simulink library "lib_transmission2"  (Simulink 4.1.1)
values from neighbouring files (symbols this model uses):
  logFlag = 1    [advSACompMaskInit.m]    (also in advSACompMaskInitR13.m)
undefined symbols (not defined in the file or in its folder): cyc_mph, fc_map_spd, fc_max_trq, fc_spd_scale, fc_trq_scale, fd_inertia, fd_loss, fd_ratio, gb_dnshift_load, gb_dnshift_spd, gb_gear_number_lookup, gb_gears_num, gb_inertia, gb_loss_const, gb_loss_input_spd_coeff, gb_loss_input_trq_coeff, gb_loss_output_spd_coeff, gb_loss_output_trq_coeff, gb_map_spd_out, gb_map_trq_in, gb_map_trq_out, gb_num_init, gb_ratio, gb_shift_delay, gb_spd_scale, gb_trq_scale, gb_upshift_load, gb_upshift_spd, htc_inertia, htc_k_adv, htc_k_adv_coast, htc_lockup, htc_lockup_load, htc_lockup_spd, htc_lu_gear_range, htc_max_coast_tr, htc_min_coast_tr, htc_pump_loss_spd, htc_pump_loss_trq_lockup, htc_pump_loss_trq_unlock, htc_sr, htc_sr_coast, htc_tr, htc_tr_coast, htc_unlock_spd, mc_map_spd, mc_max_trq, mc_overtrq_factor, mc_spd_scale, mc_trq_scale, tc_loss, tc_mc_to_fc_ratio, tx_eff_map, tx_map_spd, tx_map_trq, tx_pg_r, tx_pg_s, tx_speed_dep, vc_clutch_bool, vc_idle_spd ... (+2)
libraries: lib_controls x1, lib_etc x1, lib_controls2 x1, lib_transmission x1
(part 16 of 17)

== system lib_transmission2/Gearbox Control/automatic transmission gearbox and htc standard lockup logic for htc shift logic for gearbox/gearbox control for use w/ AT/shifting1/time since last shift ==
  in_1 : Inport  Port=1  LatchInput=off
  just shifted : Subsystem
      settings: RTWFcnNameOpts=Auto  RTWFileNameOpts=Auto
      mask Display: disp('just\nshifted')
  timer : Subsystem
      settings: RTWFcnNameOpts=Auto  RTWFileNameOpts=Auto
      mask Display: disp('timer')
  out_1 : Outport  Port=1  InitialOutput=0
  wires:
  timer/1(time) -> out_1/1
  just shifted/1(out_1) -> timer/1(trigger)
  in_1/1 -> just shifted/1(in_1)

== system lib_transmission2/Gearbox Control/automatic transmission gearbox and htc standard lockup logic for htc shift logic for gearbox/gearbox control for use w/ AT/upshift  command/load fraction ==
  In1 : Inport  Port=1  LatchInput=off
  S-Function : S-Function  FunctionName=sfun_gearbox  Parameters=load, spd  PortCounts=[]  SFunctionModules=''
  Out1 : Outport  Port=1  InitialOutput=0
  wires:
  In1/1 -> S-Function/1
  S-Function/1 -> Out1/1

== system lib_transmission2/Gearbox Control/time lookup shift logic for gearbox/lookup/shifting determination/time since last shift ==
  in_1 : Inport  Port=1  LatchInput=off
  just shifted : Subsystem
      settings: RTWFcnNameOpts=Auto  RTWFileNameOpts=Auto
      mask Display: disp('just\nshifted')
  timer : Subsystem
      settings: RTWFcnNameOpts=Auto  RTWFileNameOpts=Auto
      mask Display: disp('timer')
  out_1 : Outport  Port=1  InitialOutput=0
  wires:
  timer/1(time) -> out_1/1
  just shifted/1(out_1) -> timer/1(trigger)
  in_1/1 -> just shifted/1(in_1)

== system lib_transmission2/Gearbox Control/vehicle speed dependent shift logic for gearbox/speed dependent/Speed Dependent Shifting/shifting ==
  gear number : Inport  Port=1  LatchInput=off
  Constant : Constant  Value=gb_shift_delay-1e-6
  Relational Operator : RelationalOperator  Operator=<
  time since last shift : Subsystem
      settings: RTWFcnNameOpts=Auto  RTWFileNameOpts=Auto
      mask Display: disp('time since\nlast shift')
  out_1 : Outport  Port=1  InitialOutput=0
  wires:
  time since last shift/1(out_1) -> Relational Operator/1
  Constant/1 -> Relational Operator/2
  gear number/1 -> time since last shift/1(in_1)
  Relational Operator/1 -> out_1/1

== system lib_transmission2/Gearbox Control/vehicle speed dependent shift logic for gearbox/speed dependent/Speed Dependent Shifting/shifting1 ==
  gear number : Inport  Port=1  LatchInput=off
  Constant : Constant  Value=gb_shift_delay-1e-6
  Relational Operator : RelationalOperator  Operator=<
  time since last shift : Subsystem
      settings: RTWFcnNameOpts=Auto  RTWFileNameOpts=Auto
      mask Display: disp('time since\nlast shift')
  out_1 : Outport  Port=1  InitialOutput=0
  wires:
  time since last shift/1(out_1) -> Relational Operator/1
  Constant/1 -> Relational Operator/2
  gear number/1 -> time since last shift/1(in_1)
  Relational Operator/1 -> out_1/1

== system lib_transmission2/gearbox <gb>/gearbox model & interface/gearbox model/Pout/Pin neglecting inertia/Pout/Pin (neglecting inertia) ==
  in_1 : Inport  Port=1  LatchInput=off
  in_2 : Inport  Port=2  LatchInput=off
  Fcn : Fcn  Expr=1/u
  Product : Product  Inputs=2  Multiplication=Element-wise(.*)  SaturateOnIntegerOverflow=on
  out_1 : Outport  Port=1  InitialOutput=0
  wires:
  in_2/1 -> Fcn/1
  Product/1 -> out_1/1
  Fcn/1 -> Product/2
  in_1/1 -> Product/1

== system lib_transmission2/gearbox <gb>/gearbox model & interface/gearbox model/Pout/Pin neglecting inertia/make division bombproof ==
  note: only add eps if Tin-Tinertia is == 0 (this avoids problems when Tin-Tineratia == -eps
      | which happens from time to time
  Tin-Tinertia : Inport  Port=1  LatchInput=off
  Block NOTES : Subsystem
      settings: RTWFcnNameOpts=Auto  RTWFileNameOpts=Auto
      mask Display: disp('Block\nNOTES')
  Constant : Constant  Orientation=up  Value=eps
  Constant1 : Constant  Orientation=up  Value=0
  Product : Product  Inputs=2  Multiplication=Element-wise(.*)  SaturateOnIntegerOverflow=on
  Relational Operator1 : RelationalOperator  Operator===
  make division bombproof : Sum  Inputs=++  SaturateOnIntegerOverflow=on
  Out1 : Outport  Port=1
  wires:
  make division bombproof/1 -> Out1/1
  Constant/1 -> Product/2
  Relational Operator1/1 -> Product/1
  Product/1 -> make division bombproof/2
  Constant1/1 -> Relational Operator1/2
  Tin-Tinertia/1 -> Relational Operator1/1, make division bombproof/1

== system lib_transmission2/gearbox <gb>/gearbox model & interface/gearbox model/gearbox controller interface/enhancedToWorkspace1 ==
  In1 : Inport  Port=1  LatchInput=off
  To Workspace : ToWorkspace  VariableName=gb_gear_ratio  SampleTime=-1  SaveFormat=Array
  wires:
  In1/1 -> To Workspace/1

== system lib_transmission2/gearbox <gb>/gearbox model & interface/gearbox model/gearbox controller interface/enhancedToWorkspace8 ==
  In1 : Inport  Port=1  LatchInput=off
  To Workspace : ToWorkspace  VariableName=gb_shifting  SampleTime=-1  SaveFormat=Array
  wires:
  In1/1 -> To Workspace/1

== system lib_transmission2/gearbox <gb>/gearbox model & interface/gearbox model/loss (Nm)/3D discrete lookup table (sfun) ==
  lookup speed (rad/s) : Inport  Port=1  LatchInput=off
  lookup trq (Nm) : Inport  Port=2  LatchInput=off
  "gear_number  (e.g., 1, 2, 3)" : Inport  Port=3  LatchInput=off
  Mux : Mux  Inputs=3
  Saturation : Saturate  UpperLimit=max(tx_map_spd)  LowerLimit=min(tx_map_spd)  LinearizeAsGain=on
  Saturation1 : Saturate  UpperLimit=max(tx_map_trq)  LowerLimit=min(tx_map_trq)  LinearizeAsGain=on
  Saturation2 : Saturate  UpperLimit=size(tx_eff_map,3)  LowerLimit=1  LinearizeAsGain=on
  discrete interp2d : S-Function  FunctionName=sfun_discreteLookup3d  Parameters=tx_map_trq, tx_map_spd, tx_eff_map  PortCounts=[]  SFunctionModules=''
  tx_eff : Outport  Port=1
  wires:
  discrete interp2d/1 -> tx_eff/1
  Mux/1 -> discrete interp2d/1
  lookup speed (rad/s)/1 -> Saturation/1
  Saturation/1 -> Mux/1
  lookup trq (Nm)/1 -> Saturation1/1
  Saturation1/1 -> Mux/2
  "gear_number  (e.g., 1, 2, 3)"/1 -> Saturation2/1
  Saturation2/1 -> Mux/3

== system lib_transmission2/gearbox <gb>/gearbox model & interface/gearbox model/loss (Nm)/Block NOTES ==
  note: 5 July 2001:mpo changing loss block to a lookup table methodology
      | 12/20/00:tm revised loss saturation block. lower limit changed
      | from 1 to 0 and upper limit changed from 100 to inf to prevent over or under penalties
  note: Revision Notes:

== system lib_transmission2/gearbox <gb>/gearbox model & interface/gearbox model/loss (Nm)/enhancedToWorkspace ==
  In1 : Inport  Port=1  LatchInput=off
  To Workspace : ToWorkspace  VariableName=gb_current_gear_ratio  SampleTime=-1  SaveFormat=Array
  wires:
  In1/1 -> To Workspace/1

== system lib_transmission2/gearbox <gb>/gearbox model & interface/gearbox model/loss (Nm)/enhancedToWorkspace1 ==
  In1 : Inport  Port=1  LatchInput=off
  To Workspace : ToWorkspace  VariableName=gb_spin_loss_trq  SampleTime=-1  SaveFormat=Array
  wires:
  In1/1 -> To Workspace/1

== system lib_transmission2/gearbox <gb> CVT/CVT model & interface/CVT gearbox  <gb>/gearbox  efficiency/enhancedToWorkspace ==
  In1 : Inport  Port=1  LatchInput=off
  Terminator : Terminator
  wires:
  In1/1 -> Terminator/1

== system lib_transmission2/gearbox <gb> CVT/CVT model & interface/CVT gearbox  <gb>/loss (Nm)/Input Torque: 3-D interpolation ==
  output torque (N*m) : Inport  Port=1  LatchInput=off
  output speed (rad/s) : Inport  Port=2  LatchInput=off
  pulley ratio : Inport  Port=3  LatchInput=off
  Constant3 : Constant  Value=eps
  Constant4 : Constant  Value=0
  Demux2 : Demux  Outputs=2  BusSelectionMode=off
  Look-Up Table1 : Lookup  InputValues=[1:max(size(gb_ratio))]  OutputValues=gb_ratio
  Look-Up Table2 : Lookup  InputValues=[1:max(size(gb_ratio))]  OutputValues=gb_ratio
  Mux1 : Mux  Inputs=4
      settings: DisplayOption=none
  Mux2 : Mux  Inputs=3
      settings: DisplayOption=none
  Mux3 : Mux  Inputs=2
      settings: DisplayOption=none
  Mux4 : Mux  Inputs=2
      settings: DisplayOption=none
  Mux7 : Mux  Inputs=4
      settings: DisplayOption=none
  Product1 : Product  Inputs=3  Multiplication=Element-wise(.*)  SaturateOnIntegerOverflow=on
  Product2 : Product  Inputs=*//  Multiplication=Element-wise(.*)  SaturateOnIntegerOverflow=on
  Sum2 : Sum  Inputs=2  SaturateOnIntegerOverflow=on
  Switch1 : Switch  Threshold=eps
  indices of nearest pulley ratios for which there exist maps : Subsystem
      settings: RTWFcnNameOpts=Auto  RTWFileNameOpts=Auto
  linear eqn for power : Fcn  Expr=u[5]*(u[6]-u[3])+u[1]
  slope for linear interp. : Fcn  Expr=(u[1]-u[2])/(u[3]-u[4]+eps)
  trq in  look-up : Subsystem  mask{P1=gb_map_spd_out*gb_spd_scale, P2=gb_map_trq_in*gb_trq_scale, P3=gb_map_trq_out*gb_trq_scale, P4=gb_ratio}
      mask prompts: P1 "Vector of output speeds"; P2 "Vector of input torques"; P3 "Table of output torques"; P4 "Vector of gear ratios"
      settings: RTWFcnNameOpts=Auto  RTWFileNameOpts=Auto
  input torque (Nm) : Outport  Port=1  InitialOutput=0
  wires:
  pulley ratio/1 -> indices of nearest pulley ratios for which there exist maps/1(in_1), Mux2/3, Product2/3
  indices of nearest pulley ratios for which there exist maps/1(index of upper bounding map) -> Look-Up Table1/1, Mux7/3
  indices of nearest pulley ratios for which there exist maps/2(index of lower bounding map) -> Look-Up Table2/1, Mux7/4
  Mux7/1 -> trq in  look-up/1(In1)
  slope for linear interp./1 -> Mux2/2
  Mux2/1 -> linear eqn for power/1
  Mux1/1 -> Mux2/1, slope for linear interp./1
  Demux2/2 -> Mux1/2
  output torque (N*m)/1 -> Mux7/1
  Demux2/1 -> Mux1/1
  Look-Up Table1/1 -> Mux1/3, Mux3/1
  Look-Up Table2/1 -> Mux1/4, Mux3/2
  output speed (rad/s)/1 -> Mux7/2, Mux4/1, Mux4/2, Sum2/1, Switch1/2
  trq in  look-up/1(Out1) -> Product1/2
  Mux4/1 -> Product1/1
  Mux3/1 -> Product1/3
  Product1/1 -> Demux2/1
  linear eqn for power/1 -> Product2/1
  Sum2/1 -> Product2/2
  Product2/1 -> Switch1/1
  Switch1/1 -> input torque (Nm)/1
  Constant4/1 -> Switch1/3
  Constant3/1 -> Sum2/2

== system lib_transmission2/gearbox <gb> old/gearbox model & interface/gearbox model/Pout/Pin neglecting inertia/Pout/Pin (neglecting inertia) ==
  in_1 : Inport  Port=1  LatchInput=off
  in_2 : Inport  Port=2  LatchInput=off
  Fcn : Fcn  Expr=1/u
  Product : Product  Inputs=2  Multiplication=Element-wise(.*)  SaturateOnIntegerOverflow=on
  out_1 : Outport  Port=1  InitialOutput=0
  wires:
  in_2/1 -> Fcn/1
  Product/1 -> out_1/1
  Fcn/1 -> Product/2
  in_1/1 -> Product/1

== system lib_transmission2/gearbox <gb> old/gearbox model & interface/gearbox model/Pout/Pin neglecting inertia/make division bombproof ==
  note: only add eps if Tin-Tinertia is == 0 (this avoids problems when Tin-Tineratia == -eps
      | which happens from time to time
  Tin-Tinertia : Inport  Port=1  LatchInput=off
  Block NOTES : Subsystem
      settings: RTWFcnNameOpts=Auto  RTWFileNameOpts=Auto
      mask Display: disp('Block\nNOTES')
  Constant : Constant  Orientation=up  Value=eps
  Constant1 : Constant  Orientation=up  Value=0
  Product : Product  Inputs=2  Multiplication=Element-wise(.*)  SaturateOnIntegerOverflow=on
  Relational Operator1 : RelationalOperator  Operator===
  make division bombproof : Sum  Inputs=++  SaturateOnIntegerOverflow=on
  Out1 : Outport  Port=1
  wires:
  make division bombproof/1 -> Out1/1
  Constant/1 -> Product/2
  Relational Operator1/1 -> Product/1
  Product/1 -> make division bombproof/2
  Constant1/1 -> Relational Operator1/2
  Tin-Tinertia/1 -> Relational Operator1/1, make division bombproof/1

== system lib_transmission2/gearbox <gb> old/gearbox model & interface/gearbox model/gearbox controller interface/enhancedToWorkspace1 ==
  In1 : Inport  Port=1  LatchInput=off
  Terminator : Terminator
  wires:
  In1/1 -> Terminator/1

== system lib_transmission2/gearbox <gb> old/gearbox model & interface/gearbox model/gearbox controller interface/enhancedToWorkspace8 ==
  In1 : Inport  Port=1  LatchInput=off
  Terminator : Terminator
  wires:
  In1/1 -> Terminator/1

== system lib_transmission2/gearbox <gb> old/gearbox model & interface/gearbox model/loss (Nm)/3D discrete lookup table (sfun) ==
  lookup speed (rad/s) : Inport  Port=1  LatchInput=off
  lookup trq (Nm) : Inport  Port=2  LatchInput=off
  "gear_number  (e.g., 1, 2, 3)" : Inport  Port=3  LatchInput=off
  Mux : Mux  Inputs=3
  Saturation : Saturate  UpperLimit=max(tx_map_spd)  LowerLimit=min(tx_map_spd)  LinearizeAsGain=on
  Saturation1 : Saturate  UpperLimit=max(tx_map_trq)  LowerLimit=min(tx_map_trq)  LinearizeAsGain=on
  Saturation2 : Saturate  UpperLimit=size(tx_eff_map,3)  LowerLimit=1  LinearizeAsGain=on
  discrete interp2d : S-Function  FunctionName=sfun_discreteLookup3d  Parameters=tx_map_trq, tx_map_spd, tx_eff_map  PortCounts=[]  SFunctionModules=''
  tx_eff : Outport  Port=1
  wires:
  discrete interp2d/1 -> tx_eff/1
  Mux/1 -> discrete interp2d/1
  lookup speed (rad/s)/1 -> Saturation/1
  Saturation/1 -> Mux/1
  lookup trq (Nm)/1 -> Saturation1/1
  Saturation1/1 -> Mux/2
  "gear_number  (e.g., 1, 2, 3)"/1 -> Saturation2/1
  Saturation2/1 -> Mux/3

== system lib_transmission2/gearbox <gb> old/gearbox model & interface/gearbox model/loss (Nm)/Block NOTES ==
  note: 09/20/02:tm modifed lower input to switch after T_loss_at_input to pass the
      | total torque input as the loss when tx_eff=0
      | 5 July 2001:mpo changing loss block to a lookup table methodology
      | 12/20/00:tm revised loss saturation block. lower limit changed
      | from 1 to 0 and upper limit changed from 100 to inf to prevent over or under penalties
  note: Revision Notes:

== system lib_transmission2/gearbox <gb> old/gearbox model & interface/gearbox model/loss (Nm)/enhancedToWorkspace ==
  In1 : Inport  Port=1  LatchInput=off
  Terminator : Terminator
  wires:
  In1/1 -> Terminator/1

== system lib_transmission2/hydraulic torque converter <htc>/conventional HTC  and Interface/htc model/SR/K_adv ==
  "Req'd output trq and spd (Nm), (rad/s)" : Inport  Port=1  LatchInput=off
  >0 : Saturate  UpperLimit=inf  LowerLimit=eps  LinearizeAsGain=on
  K_adv=wout/(Tout)^0.5 : Fcn  Expr=u[2]/u[1]^0.5
  Saturation : Saturate  UpperLimit=max(htc_k_adv)  LowerLimit=min(htc_k_adv)  LinearizeAsGain=on
  K_adv : Outport  Port=1
  wires:
  >0/1 -> K_adv=wout/(Tout)^0.5/1
  "Req'd output trq and spd (Nm), (rad/s)"/1 -> >0/1
  K_adv=wout/(Tout)^0.5/1 -> Saturation/1
  Saturation/1 -> K_adv/1

== system lib_transmission2/hydraulic torque converter <htc>/conventional HTC  and Interface/htc model/SR/K_adv_coast ==
  "Req'd output trq and spd (Nm), (rad/s)" : Inport  Port=1  LatchInput=off
  K_adv=wout/(abs(Tout))^0.5 : Fcn  Expr=u[2]/abs(u[1]+eps)^0.5
  Saturation : Saturate  UpperLimit=max(htc_k_adv_coast)  LowerLimit=min(htc_k_adv_coast)  LinearizeAsGain=on
  K_adv_coast : Outport  Port=1
  wires:
  K_adv=wout/(abs(Tout))^0.5/1 -> Saturation/1
  Saturation/1 -> K_adv_coast/1
  "Req'd output trq and spd (Nm), (rad/s)"/1 -> K_adv=wout/(abs(Tout))^0.5/1

== system lib_transmission2/hydraulic torque converter <htc>/conventional HTC  and Interface/htc model/SR/enhancedToWorkspace1 ==
  In1 : Inport  Port=1  LatchInput=off
  To Workspace : ToWorkspace  VariableName=htc_coasting  SampleTime=-1  SaveFormat=Array
  wires:
  In1/1 -> To Workspace/1

== system lib_transmission2/hydraulic torque converter <htc>/conventional HTC  and Interface/htc model/SR/enhancedToWorkspace2 ==
  In1 : Inport  Port=1  LatchInput=off
  To Workspace : ToWorkspace  VariableName=htc_locked  SampleTime=-1  SaveFormat=Array
  wires:
  In1/1 -> To Workspace/1

== system lib_transmission2/hydraulic torque converter <htc>/conventional HTC  and Interface/htc model/SR/shifting SR ==
  T,w req out : Inport  Port=1  LatchInput=off
  w in : Inport  Port=2  LatchInput=off
  SR : Inport  Port=3  LatchInput=off
  -3200 rpm/second allowable in engine speed : Gain  Gain=-3200*pi/30  Multiplication=Element-wise(K.*u)  SaturateOnIntegerOverflow=on
  >0 : Saturate  UpperLimit=inf  LowerLimit=eps  LinearizeAsGain=on
  Clock : Clock
      settings: DisplayTime=off  Decimation=10
  Memory3 : Memory  X0=eps  InheritSampleTime=off
      settings: RTWStateStorageClass=Auto
  Memory4 : Memory  X0=0  InheritSampleTime=off
      settings: RTWStateStorageClass=Auto
  MinMax : MinMax  Function=min  Inputs=2
  SRmax= wout/win,min : Product  Inputs=*/  Multiplication=Element-wise(.*)  SaturateOnIntegerOverflow=on
  dt=t-(t-1) : Sum  Inputs=+-  SaturateOnIntegerOverflow=on
  "shifting, then limit  engine speed change" : Switch  Threshold=eps
  win,min= win,prev+rate*dt : Sum  Inputs=++  SaturateOnIntegerOverflow=on
  wout,req : Selector  InputType=Vector  ElementSrc=Internal  Elements=2  RowSrc=Internal  Rows=1  ColumnSrc=Internal  Columns=1  InputPortWidth=2
  SR limited : Outport  Port=1  InitialOutput=0
  wires:
  -3200 rpm/second allowable in engine speed/1 -> win,min= win,prev+rate*dt/2
  >0/1 -> Memory3/1
  w in/1 -> >0/1
  MinMax/1 -> "shifting, then limit  engine speed change"/1
  "shifting, then limit  engine speed change"/1 -> SR limited/1
  SR/1 -> MinMax/2, "shifting, then limit  engine speed change"/3
  SRmax= wout/win,min/1 -> MinMax/1
  [shifting] -> "shifting, then limit  engine speed change"/2
  T,w req out/1 -> wout,req/1
  wout,req/1 -> SRmax= wout/win,min/1
  win,min= win,prev+rate*dt/1 -> SRmax= wout/win,min/2
  Memory3/1 -> win,min= win,prev+rate*dt/1
  dt=t-(t-1)/1 -> -3200 rpm/second allowable in engine speed/1
  Clock/1 -> dt=t-(t-1)/1, Memory4/1
  Memory4/1 -> dt=t-(t-1)/2

== system lib_transmission2/hydraulic torque converter <htc>/conventional HTC  and Interface/htc model/T, shifting/T_max ==
  w_APU : Inport  Port=1  LatchInput=off
  TR : Inport  Port=2  LatchInput=off
  Saturation1 : Saturate  UpperLimit=max(fc_map_spd)*fc_spd_scale  LowerLimit=min(fc_map_spd)*fc_spd_scale  LinearizeAsGain=on
  Tin*TR= Tout : Product  Inputs=2  Multiplication=Element-wise(.*)  SaturateOnIntegerOverflow=on
  max_torque lookup : Lookup  InputValues=fc_map_spd*fc_spd_scale  OutputValues=fc_max_trq*fc_trq_scale
  T_max max gain from htc : Outport  Port=1  InitialOutput=0
  wires:
  max_torque lookup/1 -> Tin*TR= Tout/1
  TR/1 -> Tin*TR= Tout/2
  Tin*TR= Tout/1 -> T_max max gain from htc/1
  w_APU/1 -> Saturation1/1
  Saturation1/1 -> max_torque lookup/1

== system lib_transmission2/hydraulic torque converter <htc>/conventional HTC  and Interface/htc model/T, shifting/engine speed estimator ==
  htc_spd_in_a : Inport  Port=1  LatchInput=off
  Memory2 : Memory  X0=0  InheritSampleTime=off
      settings: RTWStateStorageClass=Auto
  Out1 : Outport  Port=1
  wires:
  Memory2/1 -> Out1/1
  htc_spd_in_a/1 -> Memory2/1

== system lib_transmission2/hydraulic torque converter <htc>/conventional HTC  and Interface/htc model/TR/enhancedToWorkspace2 ==
  In1 : Inport  Port=1  LatchInput=off
  To Workspace : ToWorkspace  VariableName=htc_efficiency  SampleTime=-1  SaveFormat=Array
  wires:
  In1/1 -> To Workspace/1

== system lib_transmission2/hydraulic torque converter <htc> HEV/HTC for parallel HEV and Interface/model for parallel HEV/SR/K_adv ==
  "Req'd output trq and spd (Nm), (rad/s)" : Inport  Port=1  LatchInput=off
  >0 : Saturate  UpperLimit=inf  LowerLimit=eps  LinearizeAsGain=on
  K_adv=wout/(Tout)^0.5 : Fcn  Expr=u[2]/u[1]^0.5
  Saturation : Saturate  UpperLimit=max(htc_k_adv)  LowerLimit=min(htc_k_adv)  LinearizeAsGain=on
  K_adv : Outport  Port=1
  wires:
  >0/1 -> K_adv=wout/(Tout)^0.5/1
  "Req'd output trq and spd (Nm), (rad/s)"/1 -> >0/1
  K_adv=wout/(Tout)^0.5/1 -> Saturation/1
  Saturation/1 -> K_adv/1

== system lib_transmission2/hydraulic torque converter <htc> HEV/HTC for parallel HEV and Interface/model for parallel HEV/SR/K_adv_coast ==
  "Req'd output trq and spd (Nm), (rad/s)" : Inport  Port=1  LatchInput=off
  K_adv=wout/(abs(Tout))^0.5 : Fcn  Expr=u[2]/abs(u[1]+eps)^0.5
  Saturation : Saturate  UpperLimit=max(htc_k_adv_coast)  LowerLimit=0  LinearizeAsGain=on
  K_adv_coast : Outport  Port=1
  wires:
  K_adv=wout/(abs(Tout))^0.5/1 -> Saturation/1
  Saturation/1 -> K_adv_coast/1
  "Req'd output trq and spd (Nm), (rad/s)"/1 -> K_adv=wout/(abs(Tout))^0.5/1

== system lib_transmission2/hydraulic torque converter <htc> HEV/HTC for parallel HEV and Interface/model for parallel HEV/SR/enhancedToWorkspace ==
  In1 : Inport  Port=1  LatchInput=off
  Terminator : Terminator
  wires:
  In1/1 -> Terminator/1

== system lib_transmission2/hydraulic torque converter <htc> HEV/HTC for parallel HEV and Interface/model for parallel HEV/SR/enhancedToWorkspace1 ==
  In1 : Inport  Port=1  LatchInput=off
  Terminator : Terminator
  wires:
  In1/1 -> Terminator/1

== system lib_transmission2/hydraulic torque converter <htc> HEV/HTC for parallel HEV and Interface/model for parallel HEV/SR/shifting SR ==
  T,w req out : Inport  Port=1  LatchInput=off
  w in : Inport  Port=2  LatchInput=off
  SR : Inport  Port=3  LatchInput=off
  -3200 rpm/second allowable in engine speed : Gain  Gain=-3200*pi/30  Multiplication=Element-wise(K.*u)  SaturateOnIntegerOverflow=on
  >0 : Saturate  UpperLimit=inf  LowerLimit=eps  LinearizeAsGain=on
  Clock : Clock
      settings: DisplayTime=off  Decimation=10
  Memory3 : Memory  X0=eps  InheritSampleTime=off
      settings: RTWStateStorageClass=Auto
  Memory4 : Memory  X0=0  InheritSampleTime=off
      settings: RTWStateStorageClass=Auto
  MinMax : MinMax  Function=min  Inputs=2
  SRmax= wout/win,min : Product  Inputs=*/  Multiplication=Element-wise(.*)  SaturateOnIntegerOverflow=on
  dt=t-(t-1) : Sum  Inputs=+-  SaturateOnIntegerOverflow=on
  "shifting, then limit  engine speed change" : Switch  Threshold=eps
  win,min= win,prev+rate*dt : Sum  Inputs=++  SaturateOnIntegerOverflow=on
  wout,req : Selector  InputType=Vector  ElementSrc=Internal  Elements=2  RowSrc=Internal  Rows=1  ColumnSrc=Internal  Columns=1  InputPortWidth=2
  SR limited : Outport  Port=1  InitialOutput=0
  wires:
  -3200 rpm/second allowable in engine speed/1 -> win,min= win,prev+rate*dt/2
  >0/1 -> Memory3/1
  w in/1 -> >0/1
  MinMax/1 -> "shifting, then limit  engine speed change"/1
  "shifting, then limit  engine speed change"/1 -> SR limited/1
  SR/1 -> MinMax/2, "shifting, then limit  engine speed change"/3
  SRmax= wout/win,min/1 -> MinMax/1
  [shifting] -> "shifting, then limit  engine speed change"/2
  T,w req out/1 -> wout,req/1
  wout,req/1 -> SRmax= wout/win,min/1
  win,min= win,prev+rate*dt/1 -> SRmax= wout/win,min/2
  Memory3/1 -> win,min= win,prev+rate*dt/1
  dt=t-(t-1)/1 -> -3200 rpm/second allowable in engine speed/1
  Clock/1 -> dt=t-(t-1)/1, Memory4/1
  Memory4/1 -> dt=t-(t-1)/2

== system lib_transmission2/hydraulic torque converter <htc> HEV/HTC for parallel HEV and Interface/model for parallel HEV/T, shifting/T_max ==
  w_APU : Inport  Port=1  LatchInput=off
  TR : Inport  Port=2  LatchInput=off
  Block NOTES : Subsystem
      settings: RTWFcnNameOpts=Auto  RTWFileNameOpts=Auto
      mask Display: disp('Block\nNOTES')
  Constant : Constant  Value=1
  Gain : Gain  Gain=tc_mc_to_fc_ratio  Multiplication=Element-wise(K.*u)  SaturateOnIntegerOverflow=on
  Gain1 : Gain  Gain=tc_mc_to_fc_ratio  Multiplication=Element-wise(K.*u)  SaturateOnIntegerOverflow=on
  Saturation1 : Saturate  UpperLimit=max(fc_map_spd)*fc_spd_scale  LowerLimit=min(fc_map_spd)*fc_spd_scale  LinearizeAsGain=on
  Sum : Sum  Inputs=++  SaturateOnIntegerOverflow=on
  Switch : Switch  Threshold=eps
  Tin*TR= Tout : Product  Inputs=2  Multiplication=Element-wise(.*)  SaturateOnIntegerOverflow=on
  max_torque  mc lookup1 : Lookup  InputValues=mc_map_spd*mc_spd_scale  OutputValues=mc_max_trq*mc_overtrq_factor*mc_trq_scale
  max_torque lookup : Lookup  InputValues=fc_map_spd*fc_spd_scale  OutputValues=fc_max_trq*fc_trq_scale
  T_max max gain from htc : Outport  Port=1  InitialOutput=0
  wires:
  Switch/1 -> Tin*TR= Tout/1
  Gain1/1 -> Switch/3, Sum/2
  Sum/1 -> Switch/1
  Constant/1 -> Switch/2
  max_torque  mc lookup1/1 -> Gain1/1
  Gain/1 -> max_torque  mc lookup1/1
  Saturation1/1 -> Gain/1, max_torque lookup/1
  max_torque lookup/1 -> Sum/1
  TR/1 -> Tin*TR= Tout/2
  Tin*TR= Tout/1 -> T_max max gain from htc/1
  w_APU/1 -> Saturation1/1

== system lib_transmission2/hydraulic torque converter <htc> HEV/HTC for parallel HEV and Interface/model for parallel HEV/T, shifting/engine speed estimator ==
  htc_spd_in_a : Inport  Port=1  LatchInput=off
  Memory2 : Memory  X0=0  InheritSampleTime=off
      settings: RTWStateStorageClass=Auto
  Out1 : Outport  Port=1
  wires:
  Memory2/1 -> Out1/1
  htc_spd_in_a/1 -> Memory2/1

== system lib_transmission2/hydraulic torque converter <htc> with pump loss/conventional HTC  and Interface/htc model/SR/K_adv ==
  "Req'd output trq and spd (Nm), (rad/s)" : Inport  Port=1  LatchInput=off
  >0 : Saturate  UpperLimit=inf  LowerLimit=eps  LinearizeAsGain=on
  K_adv=wout/(Tout)^0.5 : Fcn  Expr=u[2]/u[1]^0.5
  Saturation : Saturate  UpperLimit=max(htc_k_adv)  LowerLimit=min(htc_k_adv)  LinearizeAsGain=on
  K_adv : Outport  Port=1
  wires:
  >0/1 -> K_adv=wout/(Tout)^0.5/1
  "Req'd output trq and spd (Nm), (rad/s)"/1 -> >0/1
  K_adv=wout/(Tout)^0.5/1 -> Saturation/1
  Saturation/1 -> K_adv/1

== system lib_transmission2/hydraulic torque converter <htc> with pump loss/conventional HTC  and Interface/htc model/SR/K_adv_coast ==
  "Req'd output trq and spd (Nm), (rad/s)" : Inport  Port=1  LatchInput=off
  K_adv=wout/(abs(Tout))^0.5 : Fcn  Expr=u[2]/abs(u[1]+eps)^0.5
  Saturation : Saturate  UpperLimit=max(htc_k_adv_coast)  LowerLimit=min(htc_k_adv_coast)  LinearizeAsGain=on
  K_adv_coast : Outport  Port=1
  wires:
  K_adv=wout/(abs(Tout))^0.5/1 -> Saturation/1
  Saturation/1 -> K_adv_coast/1
  "Req'd output trq and spd (Nm), (rad/s)"/1 -> K_adv=wout/(abs(Tout))^0.5/1

== system lib_transmission2/hydraulic torque converter <htc> with pump loss/conventional HTC  and Interface/htc model/SR/enhancedToWorkspace1 ==
  In1 : Inport  Port=1  LatchInput=off
  To Workspace : ToWorkspace  VariableName=htc_coasting  SampleTime=-1  SaveFormat=Array
  wires:
  In1/1 -> To Workspace/1

== system lib_transmission2/hydraulic torque converter <htc> with pump loss/conventional HTC  and Interface/htc model/SR/enhancedToWorkspace2 ==
  In1 : Inport  Port=1  LatchInput=off
  To Workspace : ToWorkspace  VariableName=htc_locked  SampleTime=-1  SaveFormat=Array
  wires:
  In1/1 -> To Workspace/1

== system lib_transmission2/hydraulic torque converter <htc> with pump loss/conventional HTC  and Interface/htc model/SR/shifting SR ==
  T,w req out : Inport  Port=1  LatchInput=off
  w in : Inport  Port=2  LatchInput=off
  SR : Inport  Port=3  LatchInput=off
  -3200 rpm/second allowable in engine speed : Gain  Gain=-3200*pi/30  Multiplication=Element-wise(K.*u)  SaturateOnIntegerOverflow=on
  >0 : Saturate  UpperLimit=inf  LowerLimit=eps  LinearizeAsGain=on
  Clock : Clock
      settings: DisplayTime=off  Decimation=10
  Memory3 : Memory  X0=eps  InheritSampleTime=off
      settings: RTWStateStorageClass=Auto
  Memory4 : Memory  X0=0  InheritSampleTime=off
      settings: RTWStateStorageClass=Auto
  MinMax : MinMax  Function=min  Inputs=2
  SRmax= wout/win,min : Product  Inputs=*/  Multiplication=Element-wise(.*)  SaturateOnIntegerOverflow=on
  dt=t-(t-1) : Sum  Inputs=+-  SaturateOnIntegerOverflow=on
  "shifting, then limit  engine speed change" : Switch  Threshold=eps
  win,min= win,prev+rate*dt : Sum  Inputs=++  SaturateOnIntegerOverflow=on
  wout,req : Selector  InputType=Vector  ElementSrc=Internal  Elements=2  RowSrc=Internal  Rows=1  ColumnSrc=Internal  Columns=1  InputPortWidth=2
  SR limited : Outport  Port=1  InitialOutput=0
  wires:
  -3200 rpm/second allowable in engine speed/1 -> win,min= win,prev+rate*dt/2
  >0/1 -> Memory3/1
  w in/1 -> >0/1
  MinMax/1 -> "shifting, then limit  engine speed change"/1
  "shifting, then limit  engine speed change"/1 -> SR limited/1
  SR/1 -> MinMax/2, "shifting, then limit  engine speed change"/3
  SRmax= wout/win,min/1 -> MinMax/1
  [shifting] -> "shifting, then limit  engine speed change"/2
  T,w req out/1 -> wout,req/1
  wout,req/1 -> SRmax= wout/win,min/1
  win,min= win,prev+rate*dt/1 -> SRmax= wout/win,min/2
  Memory3/1 -> win,min= win,prev+rate*dt/1
  dt=t-(t-1)/1 -> -3200 rpm/second allowable in engine speed/1
  Clock/1 -> dt=t-(t-1)/1, Memory4/1
  Memory4/1 -> dt=t-(t-1)/2

== system lib_transmission2/hydraulic torque converter <htc> with pump loss/conventional HTC  and Interface/htc model/T, shifting/T_max ==
  w_APU : Inport  Port=1  LatchInput=off
  TR : Inport  Port=2  LatchInput=off
  Saturation1 : Saturate  UpperLimit=max(fc_map_spd)*fc_spd_scale  LowerLimit=min(fc_map_spd)*fc_spd_scale  LinearizeAsGain=on
  Tin*TR= Tout : Product  Inputs=2  Multiplication=Element-wise(.*)  SaturateOnIntegerOverflow=on
  max_torque lookup : Lookup  InputValues=fc_map_spd*fc_spd_scale  OutputValues=fc_max_trq*fc_trq_scale
  T_max max gain from htc : Outport  Port=1  InitialOutput=0
  wires:
  max_torque lookup/1 -> Tin*TR= Tout/1
  TR/1 -> Tin*TR= Tout/2
  Tin*TR= Tout/1 -> T_max max gain from htc/1
  w_APU/1 -> Saturation1/1
  Saturation1/1 -> max_torque lookup/1

== system lib_transmission2/hydraulic torque converter <htc> with pump loss/conventional HTC  and Interface/htc model/T, shifting/engine speed estimator ==
  htc_spd_in_a : Inport  Port=1  LatchInput=off
  Memory2 : Memory  X0=0  InheritSampleTime=off
      settings: RTWStateStorageClass=Auto
  Out1 : Outport  Port=1
  wires:
  Memory2/1 -> Out1/1
  htc_spd_in_a/1 -> Memory2/1

== system lib_transmission2/hydraulic torque converter <htc> with pump loss/conventional HTC  and Interface/htc model/TR/enhancedToWorkspace2 ==
  In1 : Inport  Port=1  LatchInput=off
  To Workspace : ToWorkspace  VariableName=htc_efficiency  SampleTime=-1  SaveFormat=Array
  wires:
  In1/1 -> To Workspace/1

== system lib_transmission2/hydraulic torque converter <htc> with pump loss/conventional HTC  and Interface/htc model/pump loss (Nm)/enhancedToWorkspace6 ==
  In1 : Inport  Port=1  LatchInput=off
  To Workspace : ToWorkspace  VariableName=htc_pump_loss_trq  SampleTime=-1  SaveFormat=Array
  wires:
  In1/1 -> To Workspace/1

== system lib_transmission2/Clutch Control/Clutch Control/Clutch Control/clutch control/gearbox speed estimator/Block NOTES ==
  note: The requested engine speed is replaced by an estimate of the
      | engine's previous speed whenever the vehicle missed the trace
      |  by more than 1 mph on the last time step.

== system lib_transmission2/Clutch Control/Clutch Control/Clutch Control/clutch control/gearbox speed estimator/dt ==
  Clock : Clock
      settings: DisplayTime=off  Decimation=10
  Memory1 : Memory  X0=-1  InheritSampleTime=off
      settings: RTWStateStorageClass=Auto
  Sum4 : Sum  Inputs=+-  SaturateOnIntegerOverflow=on
  Out1 : Outport  Port=1  InitialOutput=0
  wires:
  Clock/1 -> Sum4/1, Memory1/1
  Memory1/1 -> Sum4/2
  Sum4/1 -> Out1/1

== system lib_transmission2/Gearbox Control/Gearbox Control manual shift logic/manual shift logic/gearbox  control/downshift  command/load fraction ==
  In1 : Inport  Port=1  LatchInput=off
  S-Function : S-Function  FunctionName=sfun_gearbox  Parameters=load, spd  PortCounts=[]  SFunctionModules=''
  Out1 : Outport  Port=1  InitialOutput=0
  wires:
  In1/1 -> S-Function/1
  S-Function/1 -> Out1/1

== system lib_transmission2/Gearbox Control/Gearbox Control manual shift logic/manual shift logic/gearbox  control/gearbox speed estimator/Block NOTES ==
  note: The requested engine speed is replaced by an estimate of the
      | engine's previous speed whenever the vehicle missed the trace
      |  by more than 1 mph on the last time step.

== system lib_transmission2/Gearbox Control/Gearbox Control manual shift logic/manual shift logic/gearbox  control/gearbox speed estimator/dt ==
  Clock : Clock
      settings: DisplayTime=off  Decimation=10
  Memory1 : Memory  X0=-1  InheritSampleTime=off
      settings: RTWStateStorageClass=Auto
  Sum4 : Sum  Inputs=+-  SaturateOnIntegerOverflow=on
  Out1 : Outport  Port=1  InitialOutput=0
  wires:
  Sum4/1 -> Out1/1
  Memory1/1 -> Sum4/2
  Clock/1 -> Memory1/1, Sum4/1

== system lib_transmission2/Gearbox Control/Gearbox Control manual shift logic/manual shift logic/gearbox  control/shifting1/time since last shift ==
  in_1 : Inport  Port=1  LatchInput=off
  just shifted : Subsystem
      settings: RTWFcnNameOpts=Auto  RTWFileNameOpts=Auto
      mask Display: disp('just\nshifted')
  timer : Subsystem
      settings: RTWFcnNameOpts=Auto  RTWFileNameOpts=Auto
      mask Display: disp('timer')
  out_1 : Outport  Port=1  InitialOutput=0
  wires:
  in_1/1 -> just shifted/1(in_1)
  just shifted/1(out_1) -> timer/1(trigger)
  timer/1(time) -> out_1/1

== system lib_transmission2/Gearbox Control/Gearbox Control manual shift logic/manual shift logic/gearbox  control/upshift  command/load fraction ==
  In1 : Inport  Port=1  LatchInput=off
  S-Function : S-Function  FunctionName=sfun_gearbox  Parameters=load, spd  PortCounts=[]  SFunctionModules=''
  Out1 : Outport  Port=1  InitialOutput=0
  wires:
  In1/1 -> S-Function/1
  S-Function/1 -> Out1/1

== system lib_transmission2/Gearbox Control/automatic transmission gearbox and htc advanced lock-up logic for htc shift logic for gearbox/gearbox control for use w/ AT/Speed Dependent Shifting/shifting/time since last shift ==
  in_1 : Inport  Port=1  LatchInput=off
  just shifted : Subsystem
      settings: RTWFcnNameOpts=Auto  RTWFileNameOpts=Auto
      mask Display: disp('just\nshifted')
  timer : Subsystem
      settings: RTWFcnNameOpts=Auto  RTWFileNameOpts=Auto
      mask Display: disp('timer')
  out_1 : Outport  Port=1  InitialOutput=0
  wires:
  timer/1(time) -> out_1/1
  just shifted/1(out_1) -> timer/1(trigger)
  in_1/1 -> just shifted/1(in_1)

== system lib_transmission2/Gearbox Control/automatic transmission gearbox and htc advanced lock-up logic for htc shift logic for gearbox/gearbox control for use w/ AT/Speed Dependent Shifting/shifting1/time since last shift ==
  in_1 : Inport  Port=1  LatchInput=off
  just shifted : Subsystem
      settings: RTWFcnNameOpts=Auto  RTWFileNameOpts=Auto
      mask Display: disp('just\nshifted')
  timer : Subsystem
      settings: RTWFcnNameOpts=Auto  RTWFileNameOpts=Auto
      mask Display: disp('timer')
  out_1 : Outport  Port=1  InitialOutput=0
  wires:
  timer/1(time) -> out_1/1
  just shifted/1(out_1) -> timer/1(trigger)
  in_1/1 -> just shifted/1(in_1)

== system lib_transmission2/Gearbox Control/automatic transmission gearbox and htc advanced lock-up logic for htc shift logic for gearbox/gearbox control for use w/ AT/shifting1/time since last shift/just shifted ==
  in_1 : Inport  Port=1  LatchInput=off
  Memory : Memory  X0=1  InheritSampleTime=off
      settings: RTWStateStorageClass=Auto
  Relational Operator : RelationalOperator  Operator=~=
  out_1 : Outport  Port=1  InitialOutput=0
  wires:
  Relational Operator/1 -> out_1/1
  Memory/1 -> Relational Operator/1
  in_1/1 -> Relational Operator/2, Memory/1

== system lib_transmission2/Gearbox Control/automatic transmission gearbox and htc advanced lock-up logic for htc shift logic for gearbox/gearbox control for use w/ AT/shifting1/time since last shift/timer ==
  trigger : Inport  Port=1  LatchInput=off
  Constant : Constant  Value=1
  Constant1 : Constant  Value=0
  Constant2 : Constant  Value=0
  Switch : Switch  Threshold=eps
  no-lag Reset Integrator : Subsystem  mask(No-lag Reset Integrator){@1=15}
      mask prompts: @1 "Initial Value"
      mask help: No-lag Reset Integrator
      mask init:
      | initval=@1;
      settings: RTWFcnNameOpts=Auto  RTWFileNameOpts=Auto
      mask Help: Integrates first input using Euler technique.\nAt the time step that input 2 <> zero,\noutput is reset to input 3.
      mask Display: disp('1/s\nw/ reset\nno lag')
  time : Outport  Port=1  InitialOutput=0
  wires:
  Switch/1 -> time/1
  trigger/1 -> Switch/2, no-lag Reset Integrator/2(in_2)
  Constant2/1 -> Switch/1
  Constant/1 -> no-lag Reset Integrator/1(in_1)
  Constant1/1 -> no-lag Reset Integrator/3(in_3)
  no-lag Reset Integrator/1(out_1) -> Switch/3

== system lib_transmission2/Gearbox Control/automatic transmission gearbox and htc standard lockup logic for htc shift logic for gearbox/gearbox control for use w/ AT/shifting1/time since last shift/just shifted ==
  in_1 : Inport  Port=1  LatchInput=off
  Memory : Memory  X0=1  InheritSampleTime=off
      settings: RTWStateStorageClass=Auto
  Relational Operator : RelationalOperator  Operator=~=
  out_1 : Outport  Port=1  InitialOutput=0
  wires:
  in_1/1 -> Memory/1, Relational Operator/2
  Memory/1 -> Relational Operator/1
  Relational Operator/1 -> out_1/1

== system lib_transmission2/Gearbox Control/automatic transmission gearbox and htc standard lockup logic for htc shift logic for gearbox/gearbox control for use w/ AT/shifting1/time since last shift/timer ==
  trigger : Inport  Port=1  LatchInput=off
  Constant : Constant  Value=1
  Constant1 : Constant  Value=0
  Constant2 : Constant  Value=0
  Switch : Switch  Threshold=eps
  no-lag Reset Integrator : Subsystem  mask(No-lag Reset Integrator){@1=15}
      mask prompts: @1 "Initial Value"
      mask help: No-lag Reset Integrator
      mask init:
      | initval=@1;
      settings: RTWFcnNameOpts=Auto  RTWFileNameOpts=Auto
      mask Help: Integrates first input using Euler technique.\nAt the time step that input 2 <> zero,\noutput is reset to input 3.
      mask Display: disp('1/s\nw/ reset\nno lag')
  time : Outport  Port=1  InitialOutput=0
  wires:
  no-lag Reset Integrator/1(out_1) -> Switch/3
  Constant1/1 -> no-lag Reset Integrator/3(in_3)
  Constant/1 -> no-lag Reset Integrator/1(in_1)
  Constant2/1 -> Switch/1
  trigger/1 -> no-lag Reset Integrator/2(in_2), Switch/2
  Switch/1 -> time/1

== system lib_transmission2/Gearbox Control/time lookup shift logic for gearbox/lookup/shifting determination/time since last shift/just shifted ==
  in_1 : Inport  Port=1  LatchInput=off
  Memory : Memory  X0=1  InheritSampleTime=off
      settings: RTWStateStorageClass=Auto
  Relational Operator : RelationalOperator  Operator=~=
  out_1 : Outport  Port=1  InitialOutput=0
  wires:
  in_1/1 -> Memory/1, Relational Operator/2
  Memory/1 -> Relational Operator/1
  Relational Operator/1 -> out_1/1

== system lib_transmission2/Gearbox Control/time lookup shift logic for gearbox/lookup/shifting determination/time since last shift/timer ==
  trigger : Inport  Port=1  LatchInput=off
  Constant : Constant  Value=1
  Constant1 : Constant  Value=0
  Constant2 : Constant  Value=0
  Switch : Switch  Threshold=eps
  no-lag Reset Integrator : lib_controls2/<vc> conv/gearbox  control/shifting1/time since last shift/timer/no-lag Reset Integrator  MaskParam1=15
  time : Outport  Port=1  InitialOutput=0
  wires:
  no-lag Reset Integrator/1 -> Switch/3
  Constant1/1 -> no-lag Reset Integrator/3
  Constant/1 -> no-lag Reset Integrator/1
  Constant2/1 -> Switch/1
  trigger/1 -> no-lag Reset Integrator/2, Switch/2
  Switch/1 -> time/1

== system lib_transmission2/Gearbox Control/vehicle speed dependent shift logic for gearbox/speed dependent/Speed Dependent Shifting/shifting/time since last shift ==
  in_1 : Inport  Port=1  LatchInput=off
  just shifted : Subsystem
      settings: RTWFcnNameOpts=Auto  RTWFileNameOpts=Auto
      mask Display: disp('just\nshifted')
  timer : Subsystem
      settings: RTWFcnNameOpts=Auto  RTWFileNameOpts=Auto
      mask Display: disp('timer')
  out_1 : Outport  Port=1  InitialOutput=0
  wires:
  timer/1(time) -> out_1/1
  just shifted/1(out_1) -> timer/1(trigger)
  in_1/1 -> just shifted/1(in_1)

== system lib_transmission2/Gearbox Control/vehicle speed dependent shift logic for gearbox/speed dependent/Speed Dependent Shifting/shifting1/time since last shift ==
  in_1 : Inport  Port=1  LatchInput=off
  just shifted : Subsystem
      settings: RTWFcnNameOpts=Auto  RTWFileNameOpts=Auto
      mask Display: disp('just\nshifted')
  timer : Subsystem
      settings: RTWFcnNameOpts=Auto  RTWFileNameOpts=Auto
      mask Display: disp('timer')
  out_1 : Outport  Port=1  InitialOutput=0
  wires:
  timer/1(time) -> out_1/1
  just shifted/1(out_1) -> timer/1(trigger)
  in_1/1 -> just shifted/1(in_1)

== system lib_transmission2/gearbox <gb>/gearbox model & interface/gearbox model/Pout/Pin neglecting inertia/make division bombproof/Block NOTES ==
  note: this block added 10 July 2001 by mpo:
      | originally a -eps was added to the denominator by default.
      | However, cases were ecountered where Tin-Tineratia was equal to -eps causing
      | the denominator to be zero. This added checking is more rhobust

== system lib_transmission2/gearbox <gb> CVT/CVT model & interface/CVT gearbox  <gb>/loss (Nm)/Input Torque: 3-D interpolation/indices of nearest pulley ratios for which there exist maps ==
  in_1 : Inport  Port=1  LatchInput=off
  Constant : Constant  Value=1
  Look-Up Table : Lookup  InputValues=fliplr(gb_ratio)  OutputValues=fliplr([1:max(size(gb_ratio))])
  Rounding Function : Rounding  Operator=fix
  Saturation : Saturate  UpperLimit=max(size(gb_ratio))  LowerLimit=1  LinearizeAsGain=on
  Sum : Sum  Inputs=++  SaturateOnIntegerOverflow=on
  index of upper bounding map : Outport  Port=1  InitialOutput=0
  index of lower bounding map : Outport  Port=2  InitialOutput=0
  wires:
  Look-Up Table/1 -> Rounding Function/1
  in_1/1 -> Look-Up Table/1
  Constant/1 -> Sum/1
  Rounding Function/1 -> Sum/2, index of lower bounding map/1
  Saturation/1 -> index of upper bounding map/1
  Sum/1 -> Saturation/1

== system lib_transmission2/gearbox <gb> CVT/CVT model & interface/CVT gearbox  <gb>/loss (Nm)/Input Torque: 3-D interpolation/trq in  look-up ==
  In1 : Inport  Port=1  LatchInput=off
  S-Function5 : S-Function  FunctionName=sfun_gb_loss  Parameters=P1,P2,P3,P4  PortCounts=[]  SFunctionModules=''
  Out1 : Outport  Port=1  InitialOutput=0
  wires:
  S-Function5/1 -> Out1/1
  In1/1 -> S-Function5/1

== system lib_transmission2/gearbox <gb> old/gearbox model & interface/gearbox model/Pout/Pin neglecting inertia/make division bombproof/Block NOTES ==
  note: this block added 10 July 2001 by mpo:
      | originally a -eps was added to the denominator by default.
      | However, cases were ecountered where Tin-Tineratia was equal to -eps causing
      | the denominator to be zero. This added checking is more rhobust

== system lib_transmission2/hydraulic torque converter <htc> HEV/HTC for parallel HEV and Interface/model for parallel HEV/T, shifting/T_max/Block NOTES ==
  note: Notes: engine_on flag causes algebric loop. Is it necessary?
      | Doesn't seem to be. Disabled 10/31/00:tm

== system lib_transmission2/Gearbox Control/Gearbox Control manual shift logic/manual shift logic/gearbox  control/shifting1/time since last shift/just shifted ==
  in_1 : Inport  Port=1  LatchInput=off
  Memory : Memory  X0=1  InheritSampleTime=off
      settings: RTWStateStorageClass=Auto
  Relational Operator : RelationalOperator  Operator=~=
  out_1 : Outport  Port=1  InitialOutput=0
  wires:
  Relational Operator/1 -> out_1/1
  Memory/1 -> Relational Operator/1
  in_1/1 -> Relational Operator/2, Memory/1

== system lib_transmission2/Gearbox Control/Gearbox Control manual shift logic/manual shift logic/gearbox  control/shifting1/time since last shift/timer ==
  trigger : Inport  Port=1  LatchInput=off
  Constant : Constant  Value=1
  Constant1 : Constant  Value=0
  Constant2 : Constant  Value=0
  Switch : Switch  Threshold=eps
  no-lag Reset Integrator : Subsystem  mask(No-lag Reset Integrator){@1=15}
      mask prompts: @1 "Initial Value"
      mask help: No-lag Reset Integrator
      mask init:
      | initval=@1;
      settings: RTWFcnNameOpts=Auto  RTWFileNameOpts=Auto
      mask Help: Integrates first input using Euler technique.\nAt the time step that input 2 <> zero,\noutput is reset to input 3.
      mask Display: disp('1/s\nw/ reset\nno lag')
  time : Outport  Port=1  InitialOutput=0
  wires:
  Switch/1 -> time/1
  trigger/1 -> Switch/2, no-lag Reset Integrator/2(in_2)
  Constant2/1 -> Switch/1
  Constant/1 -> no-lag Reset Integrator/1(in_1)
  Constant1/1 -> no-lag Reset Integrator/3(in_3)
  no-lag Reset Integrator/1(out_1) -> Switch/3

== system lib_transmission2/Gearbox Control/automatic transmission gearbox and htc advanced lock-up logic for htc shift logic for gearbox/gearbox control for use w/ AT/Speed Dependent Shifting/shifting/time since last shift/just shifted ==
  in_1 : Inport  Port=1  LatchInput=off
  Memory : Memory  X0=1  InheritSampleTime=off
      settings: RTWStateStorageClass=Auto
  Relational Operator : RelationalOperator  Operator=~=
  out_1 : Outport  Port=1  InitialOutput=0
  wires:
  in_1/1 -> Memory/1, Relational Operator/2
  Memory/1 -> Relational Operator/1
  Relational Operator/1 -> out_1/1

== system lib_transmission2/Gearbox Control/automatic transmission gearbox and htc advanced lock-up logic for htc shift logic for gearbox/gearbox control for use w/ AT/Speed Dependent Shifting/shifting/time since last shift/timer ==
  trigger : Inport  Port=1  LatchInput=off
  Constant : Constant  Value=1
  Constant1 : Constant  Value=0
  Constant2 : Constant  Value=0
  Switch : Switch  Threshold=eps
  no-lag Reset Integrator : Subsystem  mask(No-lag Reset Integrator){@1=15}
      mask prompts: @1 "Initial Value"
      mask help: No-lag Reset Integrator
      mask init:
      | initval=@1;
      settings: RTWFcnNameOpts=Auto  RTWFileNameOpts=Auto
      mask Help: Integrates first input using Euler technique.\nAt the time step that input 2 <> zero,\noutput is reset to input 3.
      mask Display: disp('1/s\nw/ reset\nno lag')
  time : Outport  Port=1  InitialOutput=0
  wires:
  no-lag Reset Integrator/1(out_1) -> Switch/3
  Constant1/1 -> no-lag Reset Integrator/3(in_3)
  Constant/1 -> no-lag Reset Integrator/1(in_1)
  Constant2/1 -> Switch/1
  trigger/1 -> no-lag Reset Integrator/2(in_2), Switch/2
  Switch/1 -> time/1

== system lib_transmission2/Gearbox Control/automatic transmission gearbox and htc advanced lock-up logic for htc shift logic for gearbox/gearbox control for use w/ AT/Speed Dependent Shifting/shifting1/time since last shift/just shifted ==
  in_1 : Inport  Port=1  LatchInput=off
  Memory : Memory  X0=1  InheritSampleTime=off
      settings: RTWStateStorageClass=Auto
  Relational Operator : RelationalOperator  Operator=~=
  out_1 : Outport  Port=1  InitialOutput=0
  wires:
  in_1/1 -> Memory/1, Relational Operator/2
  Memory/1 -> Relational Operator/1
  Relational Operator/1 -> out_1/1

== system lib_transmission2/Gearbox Control/automatic transmission gearbox and htc advanced lock-up logic for htc shift logic for gearbox/gearbox control for use w/ AT/Speed Dependent Shifting/shifting1/time since last shift/timer ==
  trigger : Inport  Port=1  LatchInput=off
  Constant : Constant  Value=1
  Constant1 : Constant  Value=0
  Constant2 : Constant  Value=0
  Switch : Switch  Threshold=eps
  no-lag Reset Integrator : Subsystem  mask(No-lag Reset Integrator){@1=15}
      mask prompts: @1 "Initial Value"
      mask help: No-lag Reset Integrator
      mask init:
      | initval=@1;
      settings: RTWFcnNameOpts=Auto  RTWFileNameOpts=Auto
      mask Help: Integrates first input using Euler technique.\nAt the time step that input 2 <> zero,\noutput is reset to input 3.
      mask Display: disp('1/s\nw/ reset\nno lag')
  time : Outport  Port=1  InitialOutput=0
  wires:
  no-lag Reset Integrator/1(out_1) -> Switch/3
  Constant1/1 -> no-lag Reset Integrator/3(in_3)
  Constant/1 -> no-lag Reset Integrator/1(in_1)
  Constant2/1 -> Switch/1
  trigger/1 -> no-lag Reset Integrator/2(in_2), Switch/2
  Switch/1 -> time/1

== system lib_transmission2/Gearbox Control/automatic transmission gearbox and htc advanced lock-up logic for htc shift logic for gearbox/gearbox control for use w/ AT/shifting1/time since last shift/timer/no-lag Reset Integrator ==
  in_1 : Inport  Port=1  LatchInput=off
  in_2 : Inport  Port=2  LatchInput=off
  in_3 : Inport  Port=3  LatchInput=off
  Constant : Constant  Orientation=up  Value=0
  Memory : Memory  Orientation=left  X0=initval  InheritSampleTime=off
      settings: RTWStateStorageClass=Auto
  Product : Product  Inputs=2  Multiplication=Element-wise(.*)  SaturateOnIntegerOverflow=on
  Sum : Sum  Inputs=++  SaturateOnIntegerOverflow=on
  Switch : Switch  Threshold=eps
  dt : Subsystem  Orientation=down
      settings: RTWFcnNameOpts=Auto  RTWFileNameOpts=Auto
  in_2==0 : RelationalOperator  Operator===
  out_1 : Outport  Port=1  InitialOutput=0
  wires:
  in_3/1 -> Switch/3
  in_2/1 -> in_2==0/1
  in_1/1 -> Product/2
  dt/1(out_1) -> Product/1
  Product/1 -> Sum/2
  Memory/1 -> Sum/1
  Sum/1 -> Switch/1
  Switch/1 -> out_1/1, Memory/1
  in_2==0/1 -> Switch/2
  Constant/1 -> in_2==0/2
